simulink model "hw1_me451_openloop"  (R2018b)
settings: Solver=VariableStepAuto  StartTime=0.0  StopTime=10.0  RelTol=1e-3
settings Model: Creator=roone  LastModifiedBy=roone

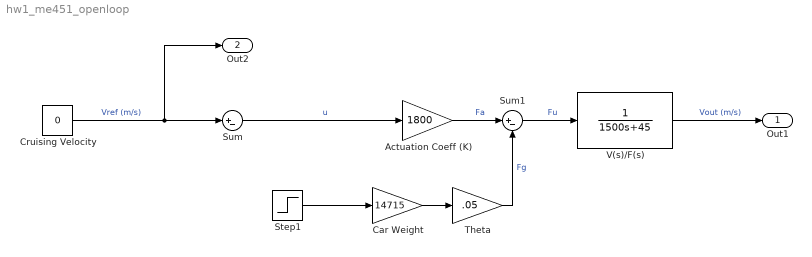
== system hw1_me451_openloop ==
  Actuation Coeff (K) : Gain  Gain=1800
  Car Weight : Gain  Gain=14715
  Cruising Velocity : Constant  Value=0
  Step1 : Step  SampleTime=0
  Sum : Sum  Inputs=|+-
  Sum1 : Sum  Inputs=|+-
  Theta : Gain  Gain=.05
  V(s)/F(s) : TransferFcn  Denominator=[1500 45]
  Out1 : Outport
  Out2 : Outport  Port=2
  wires:
  Sum/1 -> Actuation Coeff (K)/1  "u"
  Step1/1 -> Car Weight/1
  Cruising Velocity/1 -> Out2/1, Sum/1  "Vref (m/s)"
  Car Weight/1 -> Theta/1
  Actuation Coeff (K)/1 -> Sum1/1  "Fa"
  Sum1/1 -> V(s)/F(s)/1  "Fu"
  V(s)/F(s)/1 -> Out1/1  "Vout (m/s)"
  Theta/1 -> Sum1/2  "Fg"
